simulink model "F16_Real5_nn_1"  (R2013a)
settings: Solver=ode4  StartTime=0.0  StopTime=400  FixedStep=0.01  RelTol=1e-5  AbsTol=1e-4
values from neighbouring files (symbols this model uses):
  alpha0 = 1    [F16NolinearModelInitialData.m]
  altitude = 9843    [F16NolinearModelInitialData.m]
  b_ref = 9.144    [F16NolinearModelInitialData.m]
  C = [1,zeros(1,17) ... (first row only)    [F16_2003hiModelAutopilot.m]
  C2m = [C2m(1,:) ... (first row only)    [F16_2003hiModelAutopilot.m]
  dLEF = 0    [F16NolinearModelInitialData.m]
  fi_flag = 0    [F16NolinearModelInitialData.m]
  Kc = diag([0.3048,0.3048,0.3048,rad2degree,rad2degree,rad2degree,1,0.3048,rad2degree,rad2degree,rad2degree,rad2degree])    [F16InitData.m]    (also in F16InitData1.m = [1	0	0	0	0	0	0	0	0	0	0	0	0	0	0	0	0	0; F16InitData_slow.m; F16_2003hiModelAutopilot.m = [)
  Ki = [ ... (first row only)    [F16InitData.m]    (also in F16InitData_slow.m = [1.97872869	0.650510465	0; F16_2003hiModelAutopilot.m = zeros(4,3))
  Kp = [ ... (first row only)    [F16InitData.m]    (also in F16InitData_slow.m; F16_2003hiModelAutopilot.m = zeros(4,18))
  mass = 636.94*14.59428    (= 9295.6807032)    [F16NolinearModelInitialData.m]
  q = zeros(N,1)    [hose3D_n_air_Fv_correction.m]
  trim_ail = -0.01    [F16NolinearModelInitialData.m]
  trim_ele = -0.09    [F16NolinearModelInitialData.m]
  trim_rud = 0.01    [F16NolinearModelInitialData.m]
  trim_thrust = 0.17766    [F16InitData.m]    (also in F16InitData1.m = -206727.459732; F16InitData_slow.m; F16NolinearModelInitialData.m = 5000; F16_2003hiModelAutopilot.m = 2279.08519955)
undefined symbols (not defined in the file or in its folder): airSpeed, F, MIL, trim_state1
libraries: aerolibconvert2 x6, aerolibasang x4, aerolibwind2 x3, simulink x2, aerolib6dof2 x1, aerolibatmos2 x1, aerolibgravity2 x1, aerolibadyn x1
settings Model: Creator=WhisPer  LastModifiedBy=Dai

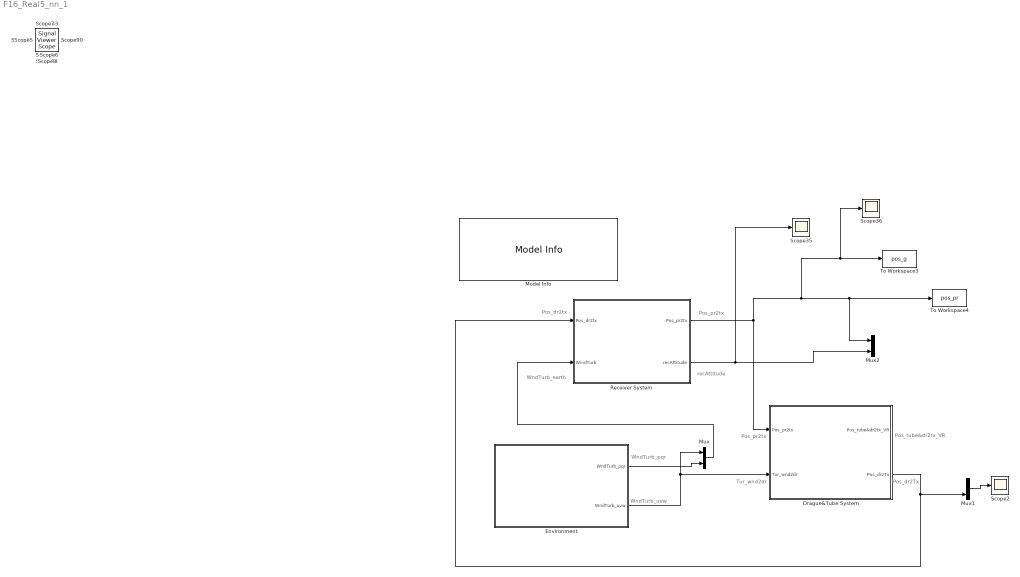
== system F16_Real5_nn_1 ==
  note: recAttitude
  note: WndTurb_uvw
  note: WndTurb_pqr
  note: Pos_dr2Tx
  note: Pos_tube&dr2tx_VR
  note: Tur_wnd2dr
  note: Pos_pr2tx
  note: WndTurb_earth
  note: Pos_dr2tx
  note: Pos_pr2tx
  Drague&Tube System : Subsystem
      mask Display: image(imread('Icon\zhuitao.png'))
  Environment : Subsystem
      mask Display: image(imread('Icon\Enviroment.jpg'))
  Model Info : simulink/Model-Wide Utilities/Model Info  InitialBlockCM=None  BlockCM=None  Frame=on  DisplayStringWithTags=|  HorizontalTextAlignment=Center  LeftAlignmentValue=0.5  SourceBlockDiagram=F16_Real5_nn_1  TagMaxNumber=20
      | Ppr_rc=[6.06 0.54 -0.86]
      | Pns_rc=[8.00 0.00  0.00]
      | Pfl_rc=[3.75 0.00 -0.86]
      | Pdr0_tk=[-13.549 0.00 5]
  Mux : Mux  Inputs=2
  Mux1 : Mux  Inputs=2
  Mux2 : Mux  Inputs=2
  Receiver System : Subsystem
      mask Display: image(imread('Icon\f16thumb.jpg'))
  Scope2 : Scope
      settings: YMin=-14  YMax=6  SaveName=ScopeData18
  Scope35 : Scope
      settings: YMin=-0.05  YMax=0.25  SaveName=ScopeData19
  Scope36 : Scope
      settings: TimeRange=20  YMin=-5.313280363223605  YMax=6.686719636776395  SaveName=ScopeData20
  To Workspace3 : ToWorkspace  VariableName=pos_g  SampleTime=-1
  To Workspace4 : ToWorkspace  VariableName=pos_pr  SampleTime=-1
  Scope{,1,3,5..9,11,13,15..34} (30 alike) : SignalViewerScope  IOType=viewer  RefreshTime=0.035000
      Scope settings: SaveName=ScopeData32
      Scope1 settings: YMin=-40  YMax=15  SaveName=ScopeData33
      Scope11 settings: SaveName=ScopeData7
      Scope13 settings: SaveName=ScopeData10
      Scope15 settings: SaveName=ScopeData12
      Scope16 settings: SaveName=ScopeData13
      Scope17 settings: SaveName=ScopeData14
      Scope18 settings: SaveName=ScopeData15
      Scope19 settings: SaveName=ScopeData16
      Scope20 settings: SaveName=ScopeData17
      Scope21 settings: SaveName=ScopeData18
      Scope22 settings: SaveName=ScopeData19
      Scope23 settings: SaveName=ScopeData20
      Scope24 settings: SaveName=ScopeData21
      Scope25 settings: SaveName=ScopeData22
      Scope26 settings: SaveName=ScopeData23
      Scope27 settings: SaveName=ScopeData24
      Scope28 settings: SaveName=ScopeData25
      Scope29 settings: SaveName=ScopeData26
      Scope3 settings: TimeRange=8  YMin=-2895.619158878505  YMax=-1095.619158878505
      Scope30 settings: SaveName=ScopeData27
      Scope31 settings: SaveName=ScopeData28
      Scope32 settings: SaveName=ScopeData29
      Scope33 settings: SaveName=ScopeData30
      Scope34 settings: YMin=-0.5  YMax=0.9  SaveName=ScopeData31
      Scope5 settings: SaveName=ScopeData2
      Scope6 settings: SaveName=ScopeData3
      Scope7 settings: SaveName=ScopeData4
      Scope8 settings: SaveName=ScopeData5
      Scope9 settings: SaveName=ScopeData9
  Scope10 : SignalViewerScope  IOType=viewer  ZoomMode=yonly  RefreshTime=0.035000
      settings: SaveName=ScopeData6
  Scope12 : SignalViewerScope  IOType=viewer  ZoomMode=xonly  RefreshTime=0.035000
      settings: SaveName=ScopeData8
  Scope14 : SignalViewerScope  IOType=viewer  ZoomMode=yonly  RefreshTime=0.035000
      settings: YMin=-1  YMax=1  SaveName=ScopeData11
  Scope4 : SignalViewerScope  IOType=viewer  ZoomMode=xonly  RefreshTime=0.035000
  wires:
  Receiver System/1(Pos_pr2tx) -> Drague&Tube System/1(Pos_pr2tx), Mux2/1, To Workspace4/1, Scope36/1, To Workspace3/1
  Drague&Tube System/2(Pos_dr2Tx) -> Receiver System/1(Pos_dr2tx), Mux1/2
  Mux/1 -> Receiver System/2(WindTurb)
  Environment/2(WndTurb_uvw) -> Drague&Tube System/2(Tur_wnd2dr), Mux/1
  Environment/1(WndTurb_pqr) -> Mux/2
  Mux1/1 -> Scope2/1
  Receiver System/2(recAttitude) -> Scope35/1, Mux2/2

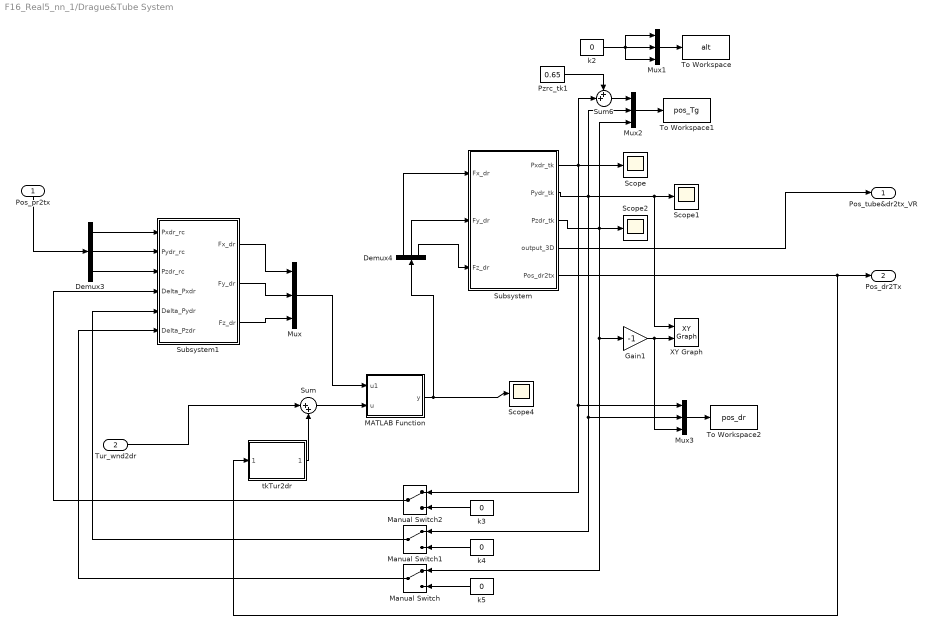
== system F16_Real5_nn_1/Drague&Tube System ==
  Pos_pr2tx : Inport
  Tur_wnd2dr : Inport  Port=2
  Demux3 : Demux  Outputs=3
  Demux4 : Demux  Outputs=3
  Gain1 : Gain  Gain=-1
  MATLAB Function : MATLAB Function  TreatAsAtomicUnit=on
  Manual Switch : ManualSwitch
  Manual Switch1 : ManualSwitch
  Manual Switch2 : ManualSwitch
  Mux{,1..3} (4 alike) : Mux  Inputs=3
  Pzrc_tk1 : Constant  Value=0.65
  Scope{,1..2,4} (4 alike) : Scope
      Scope settings: YMin=-13.32  YMax=-13.295
      Scope1 settings: YMin=-1  YMax=1
      Scope2 settings: YMin=5.155  YMax=5.22  SaveName=ScopeData2
      Scope4 settings: YMin=-2.5  YMax=47.5  SaveName=ScopeData22
  Subsystem : Subsystem
  Subsystem1 : Subsystem
  Sum : Sum  Inputs=|++
  Sum6 : Sum  Inputs=++|
  To Workspace : ToWorkspace  VariableName=alt  SampleTime=-1
  To Workspace1 : ToWorkspace  VariableName=pos_Tg  SampleTime=-1
  To Workspace2 : ToWorkspace  VariableName=pos_dr  SampleTime=-1
  XY Graph : simulink/Sinks/XY Graph  xmin=-1  xmax=1  ymin=-1-4.65  ymax=1-4.65  st=-1
  k{2..5} (4 alike) : Constant  Value=0
  tkTur2dr : MATLAB Function  TreatAsAtomicUnit=on
  Pos_tube&dr2tx_VR : Outport
  Pos_dr2Tx : Outport  Port=2
  wires:
  Demux3/2 -> Subsystem1/2(Pydr_rc)
  Demux3/3 -> Subsystem1/3(Pzdr_rc)
  Subsystem/5(Pos_dr2tx) -> tkTur2dr/1(pos_dr2tk), Pos_dr2Tx/1
  Subsystem/3(Pzdr_tk) -> Manual Switch/1, Gain1/1, Mux2/3, Scope2/1
  Gain1/1 -> Mux3/3, XY Graph/2
  Subsystem/1(Pxdr_tk) -> Mux3/1, Manual Switch2/1, Scope/1, Sum6/2
  Subsystem/2(Pydr_tk) -> Mux3/2, Manual Switch1/1, Mux2/2, XY Graph/1, Scope1/1
  Manual Switch/1 -> Subsystem1/6(Delta_Pzdr)
  Mux2/1 -> To Workspace1/1
  Mux1/1 -> To Workspace/1
  Mux3/1 -> To Workspace2/1
  k3/1 -> Manual Switch2/2
  k5/1 -> Manual Switch/2
  Pzrc_tk1/1 -> Sum6/1
  k2/1 -> Mux1/3, Mux1/1, Mux1/2
  Sum6/1 -> Mux2/1
  Manual Switch2/1 -> Subsystem1/4(Delta_Pxdr)
  Manual Switch1/1 -> Subsystem1/5(Delta_Pydr)
  k4/1 -> Manual Switch1/2
  Subsystem/4(output_3D) -> Pos_tube&dr2tx_VR/1
  Demux3/1 -> Subsystem1/1(Pxdr_rc)
  Subsystem1/1(Fx_dr) -> Mux/1
  Subsystem1/2(Fy_dr) -> Mux/2
  Sum/1 -> MATLAB Function/2(u)
  Demux4/1 -> Subsystem/1(Fx_dr)
  Demux4/2 -> Subsystem/2(Fy_dr)
  Demux4/3 -> Subsystem/3(Fz_dr)
  Subsystem1/3(Fz_dr) -> Mux/3
  Tur_wnd2dr/1 -> Sum/1
  tkTur2dr/1(TkTur2dr) -> Sum/2
  MATLAB Function/1(y) -> Scope4/1, Demux4/1
  Pos_pr2tx/1 -> Demux3/1
  Mux/1 -> MATLAB Function/1(u1)

== system F16_Real5_nn_1/Environment ==
  DCM : Constant  Value=eye(3)
  Discrete Wind Gust Model - On : aerolibwind2/Discrete Wind Gust Model  units=Metric (MKS)  Gx=on  Gy=on  Gz=on  t_0=81  d_m=[120 40 40]  v_m=[0 1 1]
  Dot Product2 : DotProduct  SaturateOnIntegerOverflow=on  OutDataTypeStr=Inherit: Inherit via internal rule
  Dryden Wind Turbulence Model (Continuous (+q -r)) : aerolibwind2/Dryden Wind Turbulence Model  (Continuous (+q -r))  units=Metric (MKS)  spec=MIL-F-8785C  model=Continuous Dryden (+q -r)  W20=5  Wdeg=0  TurbProb=10^-1  L_high=533.5  Wingspan=6  ts=0.01  Seed=1+fix(3650*rand(1,4))  T_on=on
  Length Conversion : aerolibconvert2/Length Conversion  IU=ft  OU=m
  Length Conversion1 : aerolibconvert2/Length Conversion  IU=ft  OU=m
  Sum : Sum  Inputs=+++  SaturateOnIntegerOverflow=on  InputSameDT=on  OutDataTypeStr=Inherit: Same as first input
  V2 : Math  Operator=sqrt  SaturateOnIntegerOverflow=on
  Wind Shear Model : aerolibwind2/Wind Shear Model  units=Metric (MKS)  phase=Category C - Terminal Flight Phase  W_20=1  Wdeg=0
  constan1 : Constant  Value=airSpeed
  constant : Constant  Value=altitude
  WndTurb_pqr : Outport
  WndTurb_uvw : Outport  Port=2
  wires:
  Sum/1 -> WndTurb_uvw/1
  DCM/1 -> Dryden Wind Turbulence Model (Continuous (+q -r))/3, Wind Shear Model/2
  V2/1 -> Dryden Wind Turbulence Model (Continuous (+q -r))/2, Discrete Wind Gust Model - On/1
  Dryden Wind Turbulence Model (Continuous (+q -r))/2 -> WndTurb_pqr/1
  constant/1 -> Length Conversion/1
  Dryden Wind Turbulence Model (Continuous (+q -r))/1 -> Sum/2
  Dot Product2/1 -> V2/1
  constan1/1 -> Length Conversion1/1
  Length Conversion/1 -> Dryden Wind Turbulence Model (Continuous (+q -r))/1, Wind Shear Model/1
  Length Conversion1/1 -> Dot Product2/1, Dot Product2/2

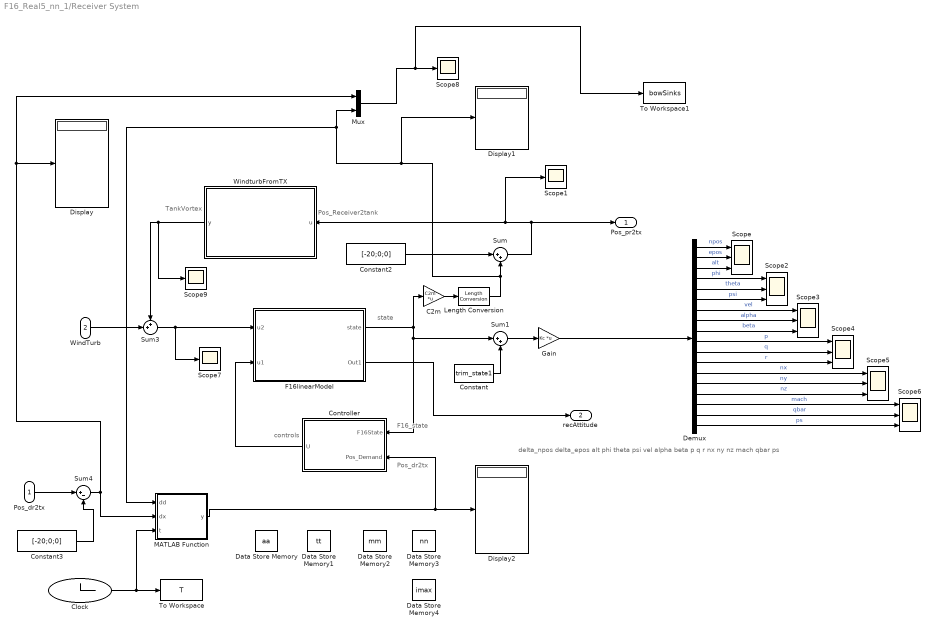
== system F16_Real5_nn_1/Receiver System ==
  note: controls
  note: Pos_dr2tx
  note: F16_state
  note: TankVortex
  note: Pos_Receiver2tank
  note: state
  note: delta_npos
      | delta_epos
      | alt
      | phi
      | theta
      | psi
      | vel
      | alpha
      | beta
      | p
      | q
      | r
      | nx
      | ny
      | nz
      | mach
      | qbar
      | ps
  Pos_dr2tx : Inport
  WindTurb : Inport  Port=2
  C2m : Gain  Gain=C2m  Multiplication=Matrix(K*u) (u vector)
  Clock : Clock
      settings: Decimation=50
  Constant : Constant  Value=trim_state1
  Constant2 : Constant  Value=[-20;0;0]
  Constant3 : Constant  Value=[-20;0;0]
  Controller : Subsystem
      mask Display: image(imread('Icon\F16_Pilot.jpg'))
  Data Store Memory : DataStoreMemory  DataStoreName=aa  InitialValue=[0;0;0]  OutDataTypeStr=double
  Data Store Memory1 : DataStoreMemory  DataStoreName=tt  OutDataTypeStr=double  Dimensions=1
  Data Store Memory2 : DataStoreMemory  DataStoreName=mm  InitialValue=[0;0.3;-0.3]  OutDataTypeStr=double
  Data Store Memory3 : DataStoreMemory  DataStoreName=nn  InitialValue=[0.2,0.1,-0.1]  OutDataTypeStr=double
  Data Store Memory4 : DataStoreMemory  DataStoreName=imax  InitialValue=[0;0]  OutDataTypeStr=double
  Demux : Demux  Outputs=18
  Display : Display
  Display1 : Display
  Display2 : Display
  F16linearModel : Subsystem
      mask Display: image(imread('Icon\fighter_f16.jpg'))
  Gain : Gain  Gain=Kc  Multiplication=Matrix(K*u) (u vector)
  Length Conversion : aerolibconvert2/Length Conversion  IU=ft  OU=m
  MATLAB Function : MATLAB Function  TreatAsAtomicUnit=on
  Mux : Mux  Inputs=2
  Scope{,2..6} (6 alike) : Scope  NumInputPorts=3
      Scope settings: YMin=-2.95~-3.2~2993.65  YMax=-1.9~-1.6~2994.13  SaveName=position  Decimation=20
      Scope2 settings: YMin=-5~-5~-5  YMax=5~5~5  SaveName=ScopeData10  Decimation=20
      Scope3 settings: YMin=119.65~0~-1.5  YMax=120.125~4~1.25  SaveName=ScopeData11  Decimation=20
      Scope4 settings: YMin=-5~-5~-5  YMax=5~5~5  SaveName=ScopeData12  Decimation=20
      Scope5 settings: YMin=-5~-5~-5  YMax=5~5~5  SaveName=ScopeData13  Decimation=20
      Scope6 settings: YMin=-5~-5~-5  YMax=5~5~5  SaveName=ScopeData5
  Scope{1,7..9} (4 alike) : Scope
      Scope1 settings: YMin=-30  YMax=10  SaveName=ScopeData7
      Scope7 settings: TimeRange=80  YMin=-1.5  SaveName=ScopeData15
      Scope8 settings: YMin=-3  YMax=7.5  SaveName=ScopeData16
      Scope9 settings: YMin=-0.25  YMax=4.5  SaveName=ScopeData21
  Sum : Sum  Inputs=|++
  Sum1 : Sum  Inputs=|++  SaturateOnIntegerOverflow=on  InputSameDT=on  OutDataTypeStr=Inherit: Same as first input
  Sum3 : Sum  Inputs=++|
  Sum4 : Sum  Inputs=|+-
  To Workspace : ToWorkspace  VariableName=T  SampleTime=-1
      settings: Decimation=100
  To Workspace1 : ToWorkspace  VariableName=bowSinks  SampleTime=-1
  WindturbFromTX : MATLAB Function  TreatAsAtomicUnit=on
  Pos_pr2tx : Outport
  recAttitude : Outport  Port=2
  wires:
  Controller/1(U) -> F16linearModel/2(u1)
  Clock/1 -> MATLAB Function/3(t), To Workspace/1
  Constant/1 -> Sum1/2
  F16linearModel/1(state) -> Controller/1(F16State), Sum1/1, C2m/1
  WindTurb/1 -> Sum3/2
  Sum1/1 -> Gain/1
  MATLAB Function/1(y) -> Controller/2(Pos_Demand), Display2/1
  Constant2/1 -> Sum/1
  Sum/1 -> Scope1/1, WindturbFromTX/1(u), Pos_pr2tx/1
  Pos_dr2tx/1 -> Sum4/1
  Sum4/1 -> Mux/1, Display/1, MATLAB Function/2(dx)
  Constant3/1 -> Sum4/2
  Mux/1 -> Scope8/1, To Workspace1/1
  WindturbFromTX/1(y) -> Sum3/1, Scope9/1
  Demux/1 -> Scope/1  "npos"
  Demux/2 -> Scope/2  "epos"
  Demux/3 -> Scope/3  "alt"
  Demux/5 -> Scope2/2  "theta"
  Demux/6 -> Scope2/3  "psi"
  Demux/7 -> Scope3/1  "vel"
  Demux/8 -> Scope3/2  "alpha"
  Demux/9 -> Scope3/3  "beta"
  Demux/10 -> Scope4/1  "p"
  Demux/11 -> Scope4/2  "q"
  Demux/12 -> Scope4/3  "r"
  Demux/13 -> Scope5/1  "nx"
  Demux/14 -> Scope5/2  "ny"
  Demux/15 -> Scope5/3  "nz"
  Demux/4 -> Scope2/1  "phi"
  Demux/16 -> Scope6/1  "mach"
  Demux/17 -> Scope6/2  "qbar"
  Demux/18 -> Scope6/3  "ps"
  Gain/1 -> Demux/1
  F16linearModel/2(Out1) -> recAttitude/1
  C2m/1 -> Length Conversion/1
  Sum3/1 -> F16linearModel/1(u2), Scope7/1
  Length Conversion/1 -> Display1/1, MATLAB Function/1(dd), Mux/2, Sum/2

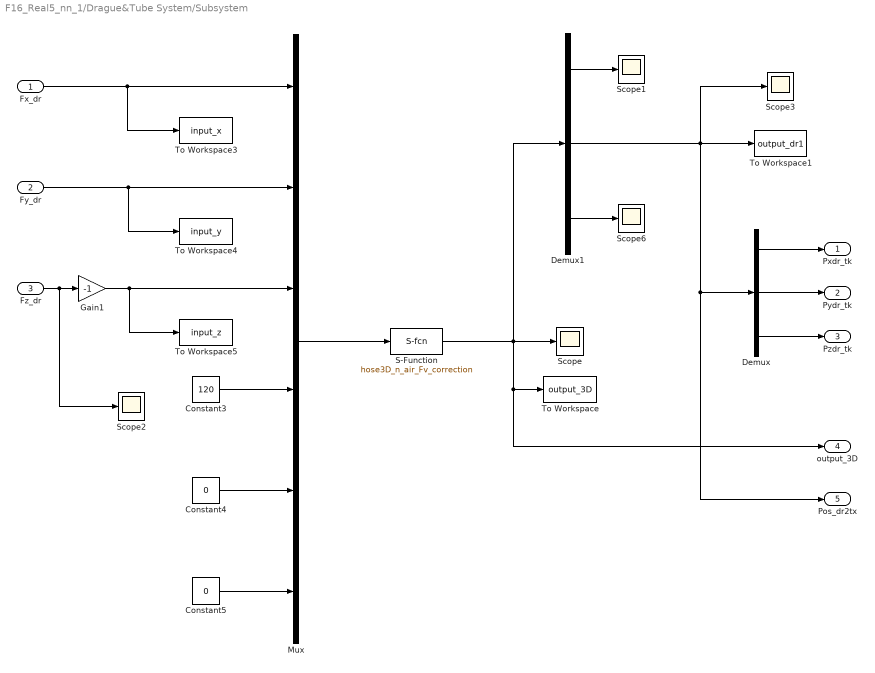
== system F16_Real5_nn_1/Drague&Tube System/Subsystem ==
  Fx_dr : Inport
  Fy_dr : Inport  Port=2
  Fz_dr : Inport  Port=3
  Constant3 : Constant  Value=120
  Constant4 : Constant  Value=0
  Constant5 : Constant  Value=0
  Demux : Demux  Outputs=3
  Demux1 : Demux  Outputs=[57,3,40]
  Gain1 : Gain  Gain=-1  ParamDataTypeStr=double  OutDataTypeStr=double
  Mux : Mux  Inputs=6
  S-Function : S-Function  FunctionName=hose3D_n_air_Fv_correction  EnableBusSupport=off
  Scope{,1..3,6} (5 alike) : Scope
      Scope settings: YMin=-14  YMax=1  SaveName=ScopeData4
      Scope1 settings: YMin=-14  YMax=1  SaveName=ScopeData3
      Scope2 settings: YMin=-65  YMax=0  SaveName=ScopeData8
      Scope3 settings: YMin=1025  YMax=1350  SaveName=ScopeData6
      Scope6 settings: YMin=-14  YMax=1  SaveName=ScopeData9
  To Workspace : ToWorkspace  VariableName=output_3D  SampleTime=-1
  To Workspace1 : ToWorkspace  VariableName=output_dr1  SampleTime=-1
  To Workspace3 : ToWorkspace  VariableName=input_x  SampleTime=-1
  To Workspace4 : ToWorkspace  VariableName=input_y  SampleTime=-1
  To Workspace5 : ToWorkspace  VariableName=input_z  SampleTime=-1
  Pxdr_tk : Outport
  Pydr_tk : Outport  Port=2
  Pzdr_tk : Outport  Port=3
  output_3D : Outport  Port=4
  Pos_dr2tx : Outport  Port=5
  wires:
  Mux/1 -> S-Function/1
  Constant3/1 -> Mux/4
  Constant4/1 -> Mux/5
  Constant5/1 -> Mux/6
  Fy_dr/1 -> Mux/2, To Workspace4/1
  Fz_dr/1 -> Scope2/1, Gain1/1
  Fx_dr/1 -> To Workspace3/1, Mux/1
  Demux1/1 -> Scope1/1
  Demux1/3 -> Scope6/1
  Demux1/2 -> Pos_dr2tx/1, Demux/1, To Workspace1/1, Scope3/1
  Demux/1 -> Pxdr_tk/1
  Demux/2 -> Pydr_tk/1
  Demux/3 -> Pzdr_tk/1
  Gain1/1 -> Mux/3, To Workspace5/1
  S-Function/1 -> Demux1/1, Scope/1, output_3D/1, To Workspace/1

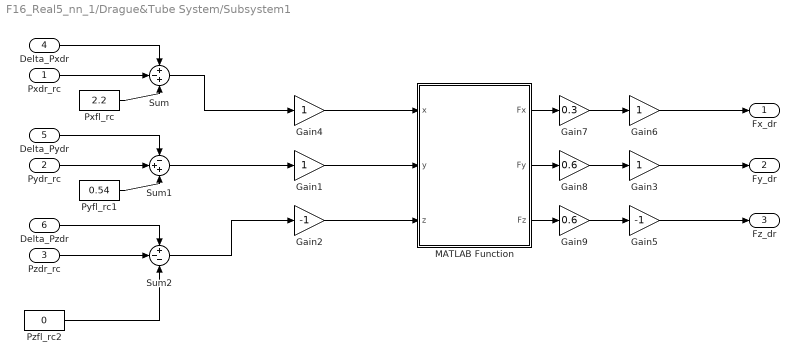
== system F16_Real5_nn_1/Drague&Tube System/Subsystem1 ==
  Pxdr_rc : Inport
  Pydr_rc : Inport  Port=2
  Pzdr_rc : Inport  Port=3
  Delta_Pxdr : Inport  Port=4
  Delta_Pydr : Inport  Port=5
  Delta_Pzdr : Inport  Port=6
  Gain{1,3..4,6} (4 alike) : Gain
  Gain2 : Gain  Gain=-1
  Gain5 : Gain  Gain=-1
  Gain7 : Gain  Gain=0.3
  Gain8 : Gain  Gain=0.6
  Gain9 : Gain  Gain=0.6
  MATLAB Function : MATLAB Function  TreatAsAtomicUnit=on
  Pxfl_rc : Constant  Value=2.2
  Pyfl_rc1 : Constant  Value=0.54
  Pzfl_rc2 : Constant  Value=0
  Sum : Sum  Inputs=+-+
  Sum1 : Sum  Inputs=-++
  Sum2 : Sum  Inputs=+--
  Fx_dr : Outport
  Fy_dr : Outport  Port=2
  Fz_dr : Outport  Port=3
  wires:
  Sum/1 -> Gain4/1
  MATLAB Function/1(Fx) -> Gain7/1
  MATLAB Function/2(Fy) -> Gain8/1
  Pxdr_rc/1 -> Sum/2
  Pxfl_rc/1 -> Sum/3
  Delta_Pxdr/1 -> Sum/1
  Pydr_rc/1 -> Sum1/2
  Delta_Pydr/1 -> Sum1/1
  Pyfl_rc1/1 -> Sum1/3
  Pzdr_rc/1 -> Sum2/2
  Pzfl_rc2/1 -> Sum2/3
  Delta_Pzdr/1 -> Sum2/1
  Gain4/1 -> MATLAB Function/1(x)
  Gain1/1 -> MATLAB Function/2(y)
  Gain2/1 -> MATLAB Function/3(z)
  Gain3/1 -> Fy_dr/1
  Gain5/1 -> Fz_dr/1
  Gain6/1 -> Fx_dr/1
  MATLAB Function/3(Fz) -> Gain9/1
  Gain7/1 -> Gain6/1
  Gain8/1 -> Gain3/1
  Gain9/1 -> Gain5/1
  Sum1/1 -> Gain1/1
  Sum2/1 -> Gain2/1

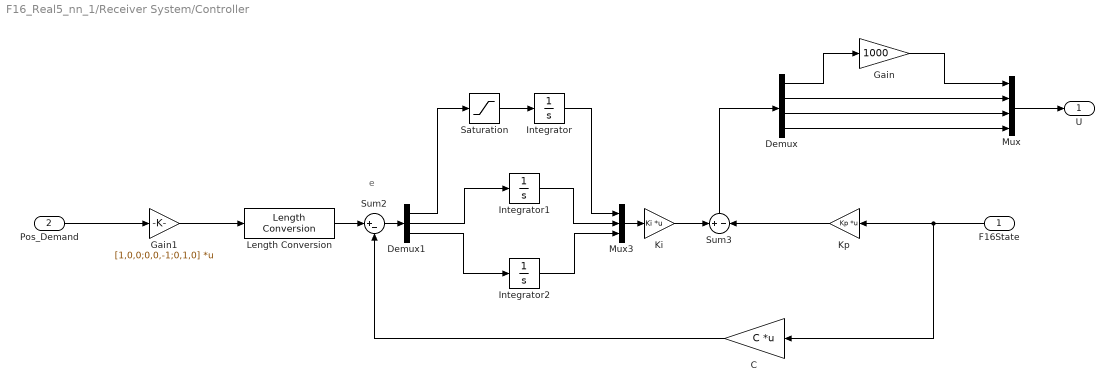
== system F16_Real5_nn_1/Receiver System/Controller ==
  note: e
  F16State : Inport
  Pos_Demand : Inport  Port=2
  C : Gain  Gain=C  Multiplication=Matrix(K*u) (u vector)
  Demux : Demux
  Demux1 : Demux  Outputs=3
  Gain : Gain  Gain=1000
  Gain1 : Gain  Gain=[1,0,0;0,0,-1;0,1,0]  Multiplication=Matrix(K*u) (u vector)
  Integrator : Integrator
  Integrator1 : Integrator
  Integrator2 : Integrator
  Ki : Gain  Gain=Ki  Multiplication=Matrix(K*u) (u vector)
  Kp : Gain  Gain=Kp  Multiplication=Matrix(K*u) (u vector)
  Length Conversion : aerolibconvert2/Length Conversion  IU=m  OU=ft
  Mux : Mux
  Mux3 : Mux  Inputs=3
  Saturation : Saturate  UpperLimit=10  LowerLimit=-10
  Sum2 : Sum  Inputs=|+-
  Sum3 : Sum  Inputs=+|-
  U : Outport
  wires:
  Sum2/1 -> Demux1/1
  C/1 -> Sum2/2
  Mux3/1 -> Ki/1
  Demux1/2 -> Integrator1/1
  F16State/1 -> Kp/1, C/1
  Integrator1/1 -> Mux3/2
  Integrator/1 -> Mux3/1
  Demux1/3 -> Integrator2/1
  Integrator2/1 -> Mux3/3
  Length Conversion/1 -> Sum2/1
  Demux1/1 -> Saturation/1
  Ki/1 -> Sum3/1
  Kp/1 -> Sum3/2
  Sum3/1 -> Demux/1
  Saturation/1 -> Integrator/1
  Demux/2 -> Mux/2
  Demux/3 -> Mux/3
  Demux/4 -> Mux/4
  Demux/1 -> Gain/1
  Gain/1 -> Mux/1
  Mux/1 -> U/1
  Pos_Demand/1 -> Gain1/1
  Gain1/1 -> Length Conversion/1

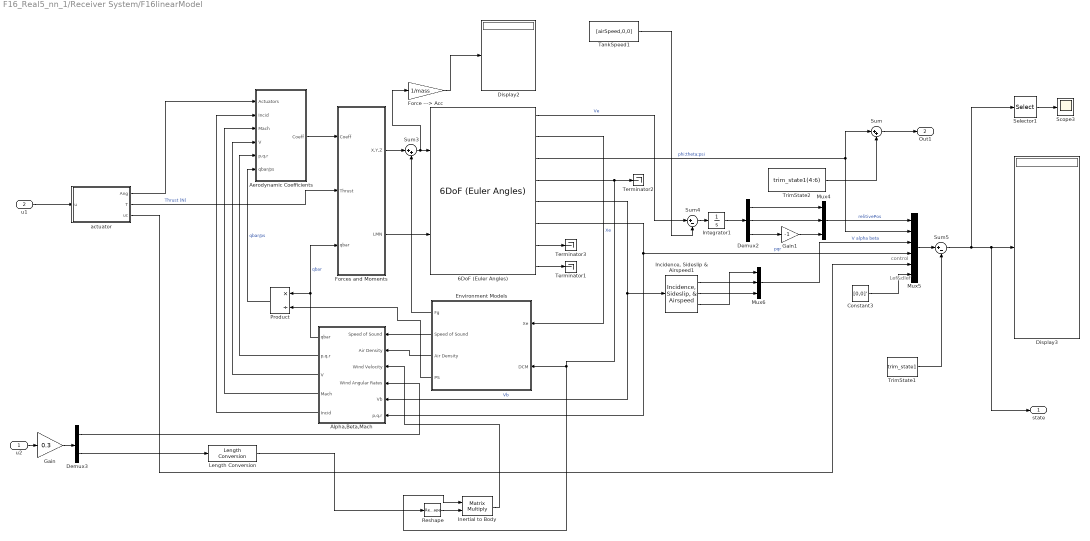
== system F16_Real5_nn_1/Receiver System/F16linearModel ==
  note: Lef&dlef
  note: control
  u2 : Inport
  u1 : Inport  Port=2
  6DoF (Euler Angles) : aerolib6dof2/6DoF (Euler Angles)  units=English (Velocity in ft/s)  mtype=Fixed  rep=Euler Angles  xme_0=xme_0  Vm_0=Vmw  eul_0=Euler_0  pm_0=pm_0  mass_0=mass  mass_e=0.5  mass_f=2.0  inertia=Inertia  inertia_e=eye(3)  inertia_f=2*eye(3)  k_quat=1.0
  Aerodynamic Coefficients : Subsystem
  Alpha,Beta,Mach : Subsystem
  Constant3 : Constant  Value=[0,0]'
  Demux2 : Demux  Outputs=3
  Demux3 : Demux  Outputs=2
  Display2 : Display
      settings: Decimation=3
  Display3 : Display
      settings: Decimation=18
  Environment Models : Subsystem
  Force ---> Acc : Gain  Gain=1/mass  SaturateOnIntegerOverflow=on  OutDataTypeStr=Inherit: Same as input  ParamDataTypeStr=Inherit: Same as input
  Forces and Moments : Subsystem
  Gain : Gain  Gain=0.3
  Gain1 : Gain  Gain=-1
  "Incidence, Sideslip & Airspeed1" : aerolibasang/Incidence, Sideslip, & Airspeed
  Inertial to Body : Product  Multiplication=Matrix(*)  SaturateOnIntegerOverflow=on  InputSameDT=on  OutDataTypeStr=Inherit: Same as first input
  Integrator1 : Integrator
  Length Conversion : aerolibconvert2/Length Conversion  IU=m  OU=ft
  Mux4 : Mux  Inputs=3
  Mux5 : Mux  Inputs=6
  Mux6 : Mux  Inputs=3
  Product : Product  Inputs=*/  SaturateOnIntegerOverflow=on  InputSameDT=on  OutDataTypeStr=Inherit: Same as first input
  Reshape : Reshape
  Scope3 : Scope
      settings: YMin=-60  YMax=10  SaveName=ScopeData14
  Selector1 : Selector  InputPortWidth=18  IndexOptions=Index vector (dialog)  Indices=[1 2 3]  OutputSizes=1
  Sum : Sum  Inputs=|++
  Sum3 : Sum  Inputs=|++  SaturateOnIntegerOverflow=on  InputSameDT=on  OutDataTypeStr=Inherit: Same as first input
  Sum4 : Sum  Inputs=|+-
  Sum5 : Sum  Inputs=|+-
  TankSpeed1 : Constant  Value=[airSpeed,0,0]
  Terminator1 : Terminator
  Terminator2 : Terminator
  Terminator3 : Terminator
  TrimState1 : Constant  Value=trim_state1
  TrimState2 : Constant  Value=trim_state1(4:6)
  actuator : Subsystem
  state : Outport
  Out1 : Outport  Port=2
  wires:
  6DoF (Euler Angles)/8 -> Terminator1/1
  6DoF (Euler Angles)/7 -> Terminator3/1
  6DoF (Euler Angles)/4 -> Inertial to Body/1, Environment Models/2(DCM), Terminator2/1
  Alpha,Beta,Mach/5(Incid) -> Aerodynamic Coefficients/2(Incid)
  Aerodynamic Coefficients/1(Coeff) -> Forces and Moments/1(Coeff)
  Environment Models/2(Speed of Sound) -> Alpha,Beta,Mach/1(Speed of Sound)
  Environment Models/3(Air Density) -> Alpha,Beta,Mach/2(Air Density)
  Forces and Moments/2(LMN) -> 6DoF (Euler Angles)/2
  Alpha,Beta,Mach/1(qbar) -> Forces and Moments/3(qbar), Product/1  "qbar"
  Forces and Moments/1(X,Y,Z) -> Sum3/1
  Sum3/1 -> Force ---> Acc/1, 6DoF (Euler Angles)/1
  Environment Models/1(Fg) -> Sum3/2
  Force ---> Acc/1 -> Display2/1
  Alpha,Beta,Mach/3(V) -> Aerodynamic Coefficients/4(V)
  Alpha,Beta,Mach/4(Mach) -> Aerodynamic Coefficients/3(Mach)
  Alpha,Beta,Mach/2("p,q,r ") -> Aerodynamic Coefficients/5(p,q,r)
  Environment Models/4(PS) -> Product/2
  Product/1 -> Aerodynamic Coefficients/6(qbar/ps)  "qbar/ps"
  u1/1 -> actuator/1(u)
  Demux3/2 -> Length Conversion/1
  Demux3/1 -> Alpha,Beta,Mach/4(Wind Angular Rates)
  actuator/2(T) -> Forces and Moments/2(Thrust)  "Thrust (N)"
  actuator/1(Ang) -> Aerodynamic Coefficients/1(Actuators)
  6DoF (Euler Angles)/3 -> Sum/1, Mux5/2  "phi;theta;psi"
  "Incidence, Sideslip & Airspeed1"/1 -> Mux6/2
  "Incidence, Sideslip & Airspeed1"/2 -> Mux6/3
  Mux6/1 -> Mux5/3  "V alpha beta"
  "Incidence, Sideslip & Airspeed1"/3 -> Mux6/1
  6DoF (Euler Angles)/6 -> Alpha,Beta,Mach/6(p,q,r), Mux5/4  "pqr"
  6DoF (Euler Angles)/5 -> Alpha,Beta,Mach/5(Vb), "Incidence, Sideslip & Airspeed1"/1  "Vb"
  Mux5/1 -> Sum5/1
  TrimState1/1 -> Sum5/2
  Sum5/1 -> state/1, Display3/1, Selector1/1
  actuator/3(uc) -> Mux5/5
  Constant3/1 -> Mux5/6
  Demux2/2 -> Mux4/2
  Demux2/3 -> Gain1/1
  Mux4/1 -> Mux5/1  "relitivePos"
  Demux2/1 -> Mux4/1
  Gain1/1 -> Mux4/3
  6DoF (Euler Angles)/1 -> Sum4/1  "Ve"
  TankSpeed1/1 -> Sum4/2
  Sum4/1 -> Integrator1/1
  Integrator1/1 -> Demux2/1
  6DoF (Euler Angles)/2 -> Environment Models/1(Xe)  "Xe"
  Selector1/1 -> Scope3/1
  u2/1 -> Gain/1
  Reshape/1 -> Inertial to Body/2
  Length Conversion/1 -> Reshape/1
  Inertial to Body/1 -> Alpha,Beta,Mach/3(Wind Velocity)
  TrimState2/1 -> Sum/2
  Sum/1 -> Out1/1
  Gain/1 -> Demux3/1

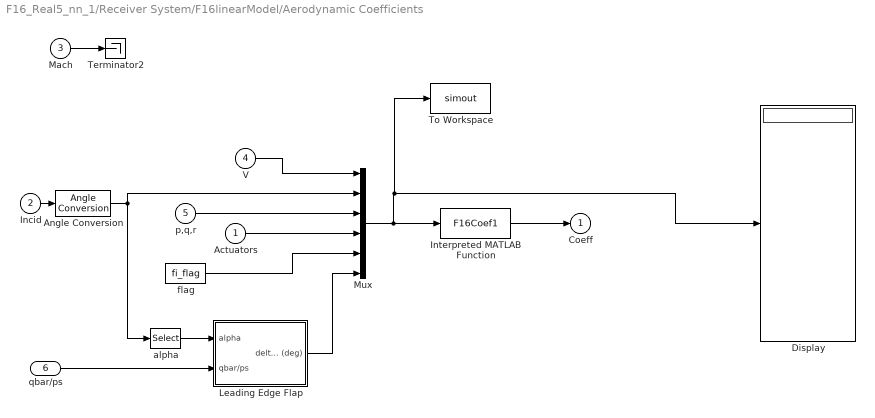
== system F16_Real5_nn_1/Receiver System/F16linearModel/Aerodynamic Coefficients ==
  Actuators : Inport
  Incid : Inport  Port=2
  Mach : Inport  Port=3
  V : Inport  Port=4
  p,q,r : Inport  Port=5
  qbar/ps : Inport  Port=6
  Angle Conversion : aerolibconvert2/Angle Conversion  IU=rad  OU=deg
  Display : Display
      settings: Decimation=12
  Interpreted MATLAB Function : MATLABFcn  MATLABFcn=F16Coef1  OutputDimensions=6
  Leading Edge Flap : Subsystem
  Mux : Mux  Inputs=6
  Terminator2 : Terminator
  To Workspace : ToWorkspace  VariableName=simout  SampleTime=-1
  alpha : Selector  InputPortWidth=2  IndexOptions=Index vector (dialog)  Indices=1  OutputSizes=1
  flag : Constant  Value=fi_flag
  Coeff : Outport  InitialOutput=0
  wires:
  Angle Conversion/1 -> alpha/1, Mux/2
  Incid/1 -> Angle Conversion/1
  qbar/ps/1 -> Leading Edge Flap/2(qbar/ps)
  alpha/1 -> Leading Edge Flap/1(alpha)
  V/1 -> Mux/1
  p,q,r/1 -> Mux/3
  Actuators/1 -> Mux/4
  flag/1 -> Mux/5
  Mach/1 -> Terminator2/1
  Interpreted MATLAB Function/1 -> Coeff/1
  Mux/1 -> To Workspace/1, Display/1, Interpreted MATLAB Function/1
  Leading Edge Flap/1(delta_lef (deg)) -> Mux/6

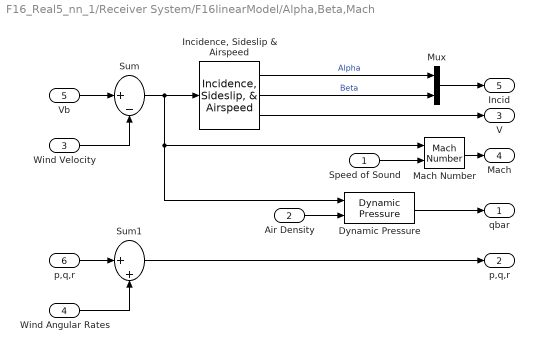
== system F16_Real5_nn_1/Receiver System/F16linearModel/Alpha,Beta,Mach ==
  Speed of Sound : Inport
  Air Density : Inport  Port=2
  Wind Velocity : Inport  Port=3  PortDimensions=3
  Wind Angular Rates : Inport  Port=4  PortDimensions=3
  Vb : Inport  Port=5  PortDimensions=3
  p,q,r : Inport  Port=6  PortDimensions=3
  Dynamic Pressure : aerolibasang/Dynamic Pressure
  "Incidence, Sideslip & Airspeed" : aerolibasang/Incidence, Sideslip, & Airspeed
  Mach Number : aerolibasang/Mach Number
  Mux : Mux  Inputs=2
  Sum : Sum  Inputs=|+-  SaturateOnIntegerOverflow=on  InputSameDT=on  OutDataTypeStr=Inherit: Same as first input
  Sum1 : Sum  Inputs=|++  SaturateOnIntegerOverflow=on  InputSameDT=on  OutDataTypeStr=Inherit: Same as first input
  qbar : Outport  InitialOutput=0
  "p,q,r " : Outport  Port=2
  V : Outport  Port=3
  Mach : Outport  Port=4
  Incid : Outport  Port=5
  wires:
  "Incidence, Sideslip & Airspeed"/3 -> V/1
  Dynamic Pressure/1 -> qbar/1
  Air Density/1 -> Dynamic Pressure/2
  Mach Number/1 -> Mach/1
  Sum/1 -> Dynamic Pressure/1, Mach Number/1, "Incidence, Sideslip & Airspeed"/1
  Vb/1 -> Sum/1
  Speed of Sound/1 -> Mach Number/2
  Wind Velocity/1 -> Sum/2
  "Incidence, Sideslip & Airspeed"/2 -> Mux/2  "Beta"
  Mux/1 -> Incid/1
  "Incidence, Sideslip & Airspeed"/1 -> Mux/1  "Alpha"
  p,q,r/1 -> Sum1/1
  Wind Angular Rates/1 -> Sum1/2
  Sum1/1 -> "p,q,r "/1

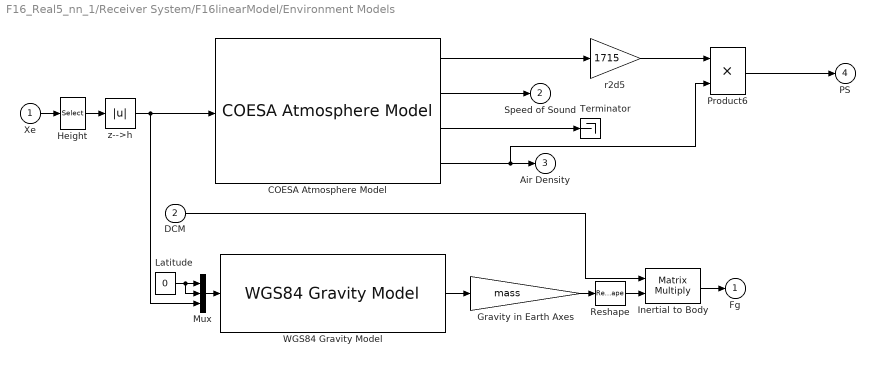
== system F16_Real5_nn_1/Receiver System/F16linearModel/Environment Models ==
  Xe : Inport  PortDimensions=3
  DCM : Inport  Port=2
  COESA Atmosphere Model : aerolibatmos2/COESA Atmosphere Model  units=English (Velocity in ft/s)  spec=1976 COESA-extended U.S. Standard Atmosphere  model=Profile  profile_var=High temperature  profile_percent=10%  profile_alt=5 km (16404 ft)  envelope_var=High temperature  envelope_percent=1%  action=None
  Gravity in Earth Axes : Gain  Gain=mass  SaturateOnIntegerOverflow=on  OutDataTypeStr=Inherit: Same as input  ParamDataTypeStr=Inherit: Same as input
  Height : Selector  InputPortWidth=3  IndexOptions=Index vector (dialog)  Indices=[3]  OutputSizes=1
  Inertial to Body : Product  Multiplication=Matrix(*)  SaturateOnIntegerOverflow=on  InputSameDT=on  OutDataTypeStr=Inherit: Same as first input
  Latitude : Constant  Value=0
  Mux : Mux  Inputs=3
  Product6 : Product  Inputs=**  SaturateOnIntegerOverflow=on  InputSameDT=on  OutDataTypeStr=Inherit: Same as first input
  Reshape : Reshape
  Terminator : Terminator
  "WGS84 Gravity Model " : aerolibgravity2/WGS84 Gravity Model   model=WGS84 Taylor Series  units=English  no_atmos=on  precessing=on  jd_loc=off  month=October  day=10  year=2004  no_centrifugal=on  action=None
  r2d5 : Gain  Gain=1715  SaturateOnIntegerOverflow=on  OutDataTypeStr=Inherit: Same as input  ParamDataTypeStr=Inherit: Same as input
  z-->h : Abs  SaturateOnIntegerOverflow=on
  Fg : Outport  InitialOutput=0
  Speed of Sound : Outport  Port=2  InitialOutput=0
  Air Density : Outport  Port=3  InitialOutput=0
  PS : Outport  Port=4
  wires:
  Reshape/1 -> Inertial to Body/2
  Mux/1 -> "WGS84 Gravity Model "/1
  z-->h/1 -> Mux/3, COESA Atmosphere Model/1
  COESA Atmosphere Model/2 -> Speed of Sound/1
  COESA Atmosphere Model/3 -> Terminator/1
  Height/1 -> z-->h/1
  Xe/1 -> Height/1
  Latitude/1 -> Mux/2, Mux/1
  "WGS84 Gravity Model "/1 -> Gravity in Earth Axes/1
  Gravity in Earth Axes/1 -> Reshape/1
  DCM/1 -> Inertial to Body/1
  Inertial to Body/1 -> Fg/1
  COESA Atmosphere Model/4 -> Product6/2, Air Density/1
  COESA Atmosphere Model/1 -> r2d5/1
  Product6/1 -> PS/1
  r2d5/1 -> Product6/1

== system F16_Real5_nn_1/Receiver System/F16linearModel/Forces and Moments ==
  Coeff : Inport
  Thrust : Inport  Port=2
  qbar : Inport  Port=3
  "Aerodynamic Forces and Moments " : aerolibadyn/Aerodynamic Forces and Moments   inputAxes=Body  outputForceAxes=Body  outputMomentAxes=Body  S=S_ref  b=b_ref  cbar=d_ref
  Center of Gravity : Constant  Value=[-0 0 0]
  Center of Pressure : Constant  Value=[-0 0 0]
  Sum : Sum  Inputs=++|  SaturateOnIntegerOverflow=on  InputSameDT=on  OutDataTypeStr=Inherit: Same as first input
  X,Y,Z : Outport  InitialOutput=0
  LMN : Outport  Port=2  InitialOutput=0
  wires:
  Center of Pressure/1 -> "Aerodynamic Forces and Moments "/4
  Center of Gravity/1 -> "Aerodynamic Forces and Moments "/3
  "Aerodynamic Forces and Moments "/1 -> Sum/2
  "Aerodynamic Forces and Moments "/2 -> LMN/1
  Sum/1 -> X,Y,Z/1
  Thrust/1 -> Sum/1
  qbar/1 -> "Aerodynamic Forces and Moments "/2
  Coeff/1 -> "Aerodynamic Forces and Moments "/1

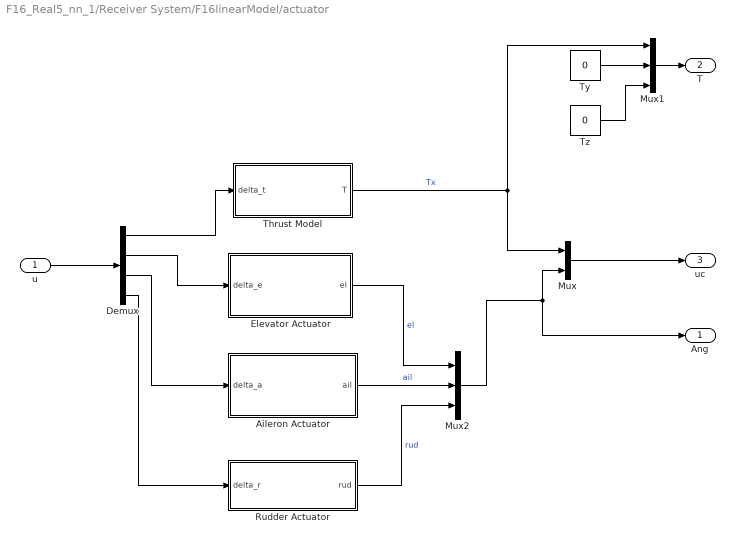
== system F16_Real5_nn_1/Receiver System/F16linearModel/actuator ==
  u : Inport
  Aileron Actuator : Subsystem
  Demux : Demux
  Elevator Actuator : Subsystem
  Mux : Mux  Inputs=2
  Mux1 : Mux  Inputs=3
  Mux2 : Mux  Inputs=3
  Rudder Actuator : Subsystem
  Thrust Model : Subsystem
  Ty : Constant  Value=0
  Tz : Constant  Value=0
  Ang : Outport
  T : Outport  Port=2
  uc : Outport  Port=3
  wires:
  u/1 -> Demux/1
  Mux2/1 -> Ang/1, Mux/2
  Thrust Model/1(T) -> Mux1/1, Mux/1  "Tx"
  Ty/1 -> Mux1/2
  Tz/1 -> Mux1/3
  Mux1/1 -> T/1
  Mux/1 -> uc/1
  Demux/1 -> Thrust Model/1(delta_t)
  Elevator Actuator/1(el) -> Mux2/1  "el"
  Aileron Actuator/1(ail) -> Mux2/2  "ail"
  Rudder Actuator/1(rud) -> Mux2/3  "rud"
  Demux/2 -> Elevator Actuator/1(delta_e)
  Demux/3 -> Aileron Actuator/1(delta_a)
  Demux/4 -> Rudder Actuator/1(delta_r)

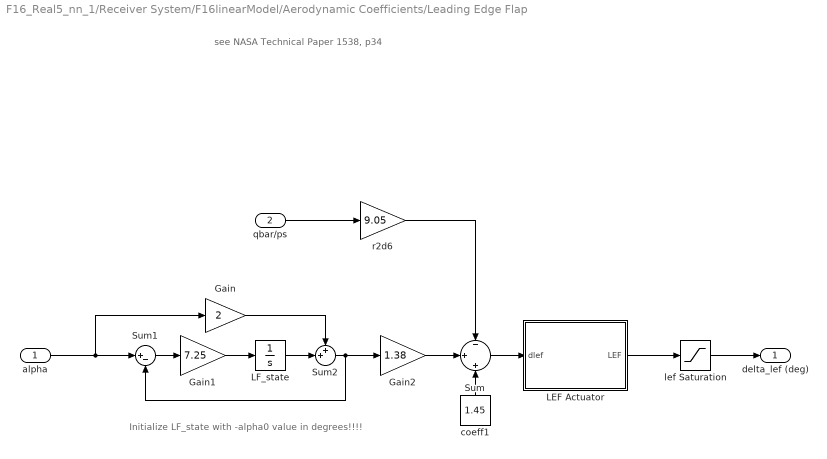
== system F16_Real5_nn_1/Receiver System/F16linearModel/Aerodynamic Coefficients/Leading Edge Flap ==
  note: see NASA Technical Paper 1538, p34
  note: Initialize LF_state with -alpha0 value in degrees!!!!
  alpha : Inport
  qbar/ps : Inport  Port=2
  Gain : Gain  Gain=2  SaturateOnIntegerOverflow=on  OutDataTypeStr=Inherit: Same as input  ParamDataTypeStr=Inherit: Same as input
  Gain1 : Gain  Gain=7.25  SaturateOnIntegerOverflow=on  OutDataTypeStr=Inherit: Same as input  ParamDataTypeStr=Inherit: Same as input
  Gain2 : Gain  Gain=1.38  SaturateOnIntegerOverflow=on  OutDataTypeStr=Inherit: Same as input  ParamDataTypeStr=Inherit: Same as input
  LEF Actuator : Subsystem
  LF_state : Integrator  InitialCondition=-alpha0
  Sum : Sum  Inputs=-|+|+  SaturateOnIntegerOverflow=on  InputSameDT=on  OutDataTypeStr=Inherit: Same as first input
  Sum1 : Sum  Inputs=|+-  SaturateOnIntegerOverflow=on  InputSameDT=on  OutDataTypeStr=Inherit: Same as first input
  Sum2 : Sum  Inputs=++|  SaturateOnIntegerOverflow=on  InputSameDT=on  OutDataTypeStr=Inherit: Same as first input
  coeff1 : Constant  Value=1.45
  lef Saturation : Saturate  UpperLimit=25  LowerLimit=0
  r2d6 : Gain  Gain=9.05  SaturateOnIntegerOverflow=on  OutDataTypeStr=Inherit: Same as input  ParamDataTypeStr=Inherit: Same as input
  delta_lef (deg) : Outport
  wires:
  Sum1/1 -> Gain1/1
  Gain1/1 -> LF_state/1
  Gain/1 -> Sum2/1
  Gain2/1 -> Sum/2
  coeff1/1 -> Sum/3
  Sum2/1 -> Sum1/2, Gain2/1
  LF_state/1 -> Sum2/2
  alpha/1 -> Sum1/1, Gain/1
  qbar/ps/1 -> r2d6/1
  r2d6/1 -> Sum/1
  lef Saturation/1 -> delta_lef (deg)/1
  Sum/1 -> LEF Actuator/1(dlef)
  LEF Actuator/1(LEF) -> lef Saturation/1

== system F16_Real5_nn_1/Receiver System/F16linearModel/actuator/Aileron Actuator ==
  delta_a : Inport
  Command Saturation : Saturate  UpperLimit=21.5  LowerLimit=-21.5
  Gain : Gain  Gain=20.2  SaturateOnIntegerOverflow=on  OutDataTypeStr=Inherit: Same as input  ParamDataTypeStr=Inherit: Same as input
  "Integrator " : Integrator  InitialCondition=trim_ail  UpperSaturationLimit=21.5  LowerSaturationLimit=-21.5
  Rate Saturation : Saturate  UpperLimit=80  LowerLimit=-80
  Sum : Sum  Inputs=|+-  SaturateOnIntegerOverflow=on  InputSameDT=on  OutDataTypeStr=Inherit: Same as first input
  ail : Outport
  wires:
  delta_a/1 -> Command Saturation/1
  "Integrator "/1 -> ail/1, Sum/2
  Sum/1 -> Gain/1
  Gain/1 -> Rate Saturation/1
  Command Saturation/1 -> Sum/1
  Rate Saturation/1 -> "Integrator "/1

== system F16_Real5_nn_1/Receiver System/F16linearModel/actuator/Elevator Actuator ==
  delta_e : Inport
  Command Saturation : Saturate  UpperLimit=25  LowerLimit=-25
  Gain : Gain  Gain=20.2  SaturateOnIntegerOverflow=on  OutDataTypeStr=Inherit: Same as input  ParamDataTypeStr=Inherit: Same as input
  "Integrator " : Integrator  InitialCondition=trim_ele  UpperSaturationLimit=25  LowerSaturationLimit=-25
  Rate Saturation : Saturate  UpperLimit=60  LowerLimit=-60
  Sum : Sum  Inputs=|+-  SaturateOnIntegerOverflow=on  InputSameDT=on  OutDataTypeStr=Inherit: Same as first input
  el : Outport
  wires:
  delta_e/1 -> Command Saturation/1
  Command Saturation/1 -> Sum/1
  Sum/1 -> Gain/1
  Gain/1 -> Rate Saturation/1
  "Integrator "/1 -> el/1, Sum/2
  Rate Saturation/1 -> "Integrator "/1

== system F16_Real5_nn_1/Receiver System/F16linearModel/actuator/Rudder Actuator ==
  delta_r : Inport
  Command Saturation : Saturate  UpperLimit=30  LowerLimit=-30
  Gain : Gain  Gain=20.2  SaturateOnIntegerOverflow=on  OutDataTypeStr=Inherit: Same as input  ParamDataTypeStr=Inherit: Same as input
  "Integrator " : Integrator  InitialCondition=trim_rud  UpperSaturationLimit=30  LowerSaturationLimit=-30
  Rate Saturation : Saturate  UpperLimit=120  LowerLimit=-120
  Sum : Sum  Inputs=|+-  SaturateOnIntegerOverflow=on  InputSameDT=on  OutDataTypeStr=Inherit: Same as first input
  rud : Outport
  wires:
  "Integrator "/1 -> rud/1, Sum/2
  Sum/1 -> Gain/1
  delta_r/1 -> Command Saturation/1
  Rate Saturation/1 -> "Integrator "/1
  Gain/1 -> Rate Saturation/1
  Command Saturation/1 -> Sum/1

== system F16_Real5_nn_1/Receiver System/F16linearModel/actuator/Thrust Model ==
  delta_t : Inport
  Command Saturation : Saturate  UpperLimit=19000  LowerLimit=1000
  Gain : Gain  SaturateOnIntegerOverflow=on  OutDataTypeStr=Inherit: Same as input  ParamDataTypeStr=Inherit: Same as input
  "Integrator " : Integrator  InitialCondition=trim_thrust  UpperSaturationLimit=30  LowerSaturationLimit=-30
  Rate Saturation : Saturate  UpperLimit=10000  LowerLimit=-10000
  Sum : Sum  Inputs=|+-  SaturateOnIntegerOverflow=on  InputSameDT=on  OutDataTypeStr=Inherit: Same as first input
  T : Outport
  wires:
  delta_t/1 -> Command Saturation/1
  Gain/1 -> Rate Saturation/1
  "Integrator "/1 -> T/1, Sum/2
  Command Saturation/1 -> Sum/1
  Sum/1 -> Gain/1
  Rate Saturation/1 -> "Integrator "/1

== system F16_Real5_nn_1/Receiver System/F16linearModel/Aerodynamic Coefficients/Leading Edge Flap/LEF Actuator ==
  dlef : Inport
  Command Saturation : Saturate  UpperLimit=25  LowerLimit=0
  Gain3 : Gain  Gain=1/0.136  SaturateOnIntegerOverflow=on  OutDataTypeStr=Inherit: Same as input  ParamDataTypeStr=Inherit: Same as input
  "Integrator " : Integrator  InitialCondition=dLEF  UpperSaturationLimit=21.5  LowerSaturationLimit=-21.5
  Rate Saturation : Saturate  UpperLimit=25  LowerLimit=-25
  Sum3 : Sum  Inputs=|+-  SaturateOnIntegerOverflow=on  InputSameDT=on  OutDataTypeStr=Inherit: Same as first input
  LEF : Outport
  wires:
  Gain3/1 -> Rate Saturation/1
  Rate Saturation/1 -> "Integrator "/1
  "Integrator "/1 -> LEF/1, Sum3/2
  Sum3/1 -> Gain3/1
  dlef/1 -> Command Saturation/1
  Command Saturation/1 -> Sum3/1

== matlab function F16_Real5_nn_1/Receiver System/MATLAB Function ==
  data: dd input; dx input; y output; t input; aa data_store_memory; tt data_store_memory; mm data_store_memory; nn data_store_memory; imax data_store_memory
function y = fcn(dd,dx,t)
%#codegen
%输入为xd，yd,-h
%调整为xd,h,yd

global aa;
global tt;
global mm;
global nn;
global imax;

t1=t-tt;
if t1<20
   y=[0;-2;6] ;
elseif t1<50
     y=[4;dx(2);dx(3)];  
     if t1>44&&t1<45
        aa=y; 
     end
     if t1>45
         aa=1/3*aa+2/3*y;           %;做一个滤波，求出锥套的平衡点。
     end 
     if t>50&&t1>20&&t1<23
         y=[2;0;6];
     end
          
else
    deltaX=dd(1)-dx(1);
    if deltaX<-1 || deltaX>0
        nz=0;
        ny=0;
    else
        nz=1*(1-deltaX^2);
        ny=1*(1-deltaX^2);
    end
    %dx

    y=[dx(1)+nn(1);(1-ny)*(aa(2)+mm(2)+nn(2))+ny*(dx(2));(1-nz)*(aa(3)+mm(3)+nn(3))+nz*(dx(3))];
    
    %y=[dx(1)+nn(1);aa(2)+mm(2)+nn(2);aa(3)+mm(3)+nn(3)];
    %y=dx;
    if abs(dd(1)-dx(1))<0.01
       tt=t-21; 
       %mm=1/2*mm+1/2*[0;(dx(2)-aa(2));(dx(3)-aa(3))];%+1/3*[0;(dx(2)-dd(2));-(dx(3)-dd(3))];
       mm=1/2*mm+1/2*[0;imax(1);imax(2)];
       
       nn=nn+0.75*[0;(dx(2)-dd(2));(dx(3)-dd(3))];
       imax=[0;0];
    else
       if abs(dx(2)-aa(2))>abs(imax(1))
            nn(2)=dx(2)-aa(2);
       end
       if abs(dx(3)-aa(3))>abs(imax(2))
            imax(2)=dx(3)-aa(3);
       end       
    end

end

% global aa;
% global tt;
% global mm;
% global nn;
% 
% t1=t-tt;
% 
% if t1<50
%      y=[2;dx(2);dx(3)];  
%      if t1>44&&t1<45
%         aa=y; 
%      end
%      if t1>45
%          aa=1/3*aa+2/3*y;           %;做一个滤波，求出锥套的平衡点。
%      end
%      
%      if t>50&&t1>20&&t1<23
%          y=[2;aa(2);aa(3)];
%      end
%      
% else
%     deltaX=dd(1)-dx(1);
%     if deltaX<-1 || deltaX>0
%         nz=0;
%         ny=0;
%     elseif deltaX>-0.5
%         nz=1;
%         ny=1;
%     else
%         nz=2*(1-deltaX^2);
%         ny=2*(1-deltaX^2);
%     end
%     %dx
%     y=[dx(1)+nn(1);(1-ny)*(dx(2)+nn(2))+ny*(dx(2));(1-nz)*(dx(3)+nn(3))+nz*(dx(3))];
%     
%     %y=dx;
%     if abs(deltaX)<0.01
%        tt=t-20; 
%        mm=1/2*mm+1/2*[0;nn(2);nn(3)];%+1/3*[0;(dx(2)-dd(2));-(dx(3)-dd(3))];
%        nn=nn+1/2*[0;(dx(2)-dd(2));(dx(3)-dd(3))];
%        
%        %nn=nn+1/3*[0;(dx(2)-dd(2));(dx(3)-dd(3))]; 
% %        nn(2)=0.1;nn(3)=-0.1;
% %     else
% %        if abs(dx(2)-aa(2))>abs(nn(2))
% %             nn(2)=dx(2)-aa(2);
% %        end
% %        if abs(dx(3)-aa(3))>abs(nn(3))
% %             nn(3)=dx(3)-aa(3);
% %        end
%     end
% 
% end


% 
% dx=[dx(1);dx(2);dx(3)];
% dd=[dd(1);dd(2);dd(3)];
% 
% t1=t-tt;
% % if t<5
% %     y=[2;-10;-4];
% % elseif t<10
% %     y=[1;10;4];
% % elseif t<20
% %     y=[4;-10;-4];
% if t1<20
%     y=[0;-6;-2];
% elseif t1<50
%      y=[4;dx(2);dx(3)];  
%      if t1>44&&t1<45
%         aa=y; 
%      end
%      if t1>45
%          aa=1/3*aa+2/3*y           %;做一个滤波，求出锥套的平衡点。
%      end
% else
%     y=[dx(1);aa(2)+mm(2);aa(3)+mm(3)];
%     %y=dx;
%     if abs(dd(1)-dx(1))<0.01
%        tt=t-21; 
%        mm=1/3*mm+2/3*[0;(aa(2)-dd(2));-(aa(3)-dd(3))]%+1/3*[0;(dx(2)-dd(2));-(dx(3)-dd(3))];
%     end
%         
% end

== matlab function F16_Real5_nn_1/Drague&Tube System/Subsystem1/MATLAB Function ==
  data: x input; Fx output; y input; z input; Fy output; Fz output
function [Fx,Fy,Fz] = F_rc2dr(x,y,z)

% Fz = 229.5*(1-0.2122*x)*exp(-y^2/0.5341)*exp(-z/0.7166)*(0.5-1/pi*atan(1000*(x-4.71)));
% Fy = 330.9*(1-0.2181*x)*(y*exp(-y^2/0.878))*exp(-z/0.5684)*(0.5-1/pi*atan(1000*(x-4.615)));
% Fx = 121.2224*(1-0.3918*(x-3.9316)^2)*exp(-y^2/2.226)*exp(-z/1.673)*(0.5-1/pi*atan(1000*(x-5.55)))...
%                     +519*(1-0.325*x)*exp(-y^2/0.5599)*exp(-z/0.8122)*(0.5-1/pi*atan(1000*(x-3.048)));

if x > 1/0.2161
    Fz = 0;
else
    Fz = 174.0219*(1-0.2161*x)*exp(-y^2/0.5862)*exp(-z/0.6364);
end

if x > 1/0.2128
    Fy = 0;
else
    Fy = 223.4144*(1-0.2128*x)*(y*exp(-y^2/0.8480))*exp(-z/0.6874);
end

if x > sqrt(1/0.3774)+3.9471
    Fx = 0;
elseif x > 1/0.3149
    Fx = 92.0795*(1-0.3774*(x-3.9471)^2)*exp(-y^2/2.6073)*exp(-z/1.5244);
else
    Fx = 92.0795*(1-0.3774*(x-3.9471)^2)*exp(-y^2/2.6073)*exp(-z/1.5244)...
                 + 338.6175*(1-0.3149*x)*exp(-y^2/0.4435)*exp(-z/1.0890);
end

== matlab function F16_Real5_nn_1/Drague&Tube System/MATLAB Function ==
  data: u1 input; u input; y output
function y = Dr_wnd2Frc(u1,u)
%#codegen

Ve=120;
rho = 0.98;
Q=0.5*rho*Ve^2;
S=0.38;
CD=0.81*0.8;

uu=u(1);
vv=u(2);
ww=u(3);

%beta = acos(sqrt(vv^2+ww^2)/abs(uu));
%theta = atan(ww/vv);

C_beta = 0.3979;

yx=rho*S*CD*Ve*uu;
yy=Q*S*C_beta*vv/Ve;
yz=Q*S*C_beta*ww/Ve;


y = [yx,yy,yz]';
y=u1+y;

== matlab function F16_Real5_nn_1/Receiver System/WindturbFromTX ==
  data: u input; y output
function y = WindTurFromTank(u)
%#codegen

%横纵向气流角速度等下计算长度
c_lat=4;
c_lon=4;

%两端参考点
u1 = u+[0 ,c_lat ,0]';
u2 = u+[0 ,-c_lat, 0]';

yy1 = TankerVortexWindField(u1);
yy2 = TankerVortexWindField(u2);

%计算x轴向滚转角速度
yp = (yy1(3) - yy2(3))/4/c_lat;

u3=u+[c_lon, 0,0]';
u4=u+[-c_lon ,0,0]';
yy3 = TankerVortexWindField(u3);
yy4 = TankerVortexWindField(u4);

%俯仰角速度计算
yq = -(yy3(3) - yy4(3))/4/c_lon;

%偏航角速度设为0
yr = 0;

%质心处风场计算
y_uvw = TankerVortexWindField(u);


%y = [y_uvw(1);y_uvw(2);y_uvw(3);-yp;-yq;-yr]*0.5;
y = [y_uvw(1);y_uvw(2);y_uvw(3);-yp;-yq;-yr];

== matlab function F16_Real5_nn_1/Drague&Tube System/tkTur2dr ==
  data: pos_dr2tk input; TkTur2dr output
function TkTur2dr = fcn(pos_dr2tk)
%#codegen

TkTur2dr = TankerVortexWindField(pos_dr2tk);
